simulink model "grav"  (R2017b)
settings: Solver=ode5  StartTime=0.0  StopTime=5*86400  FixedStep=60  RelTol=1e-3
undefined symbols (not defined in the file): Cube, G
settings Model: Creator=hazr_sh  LastModifiedBy=shriyahazra

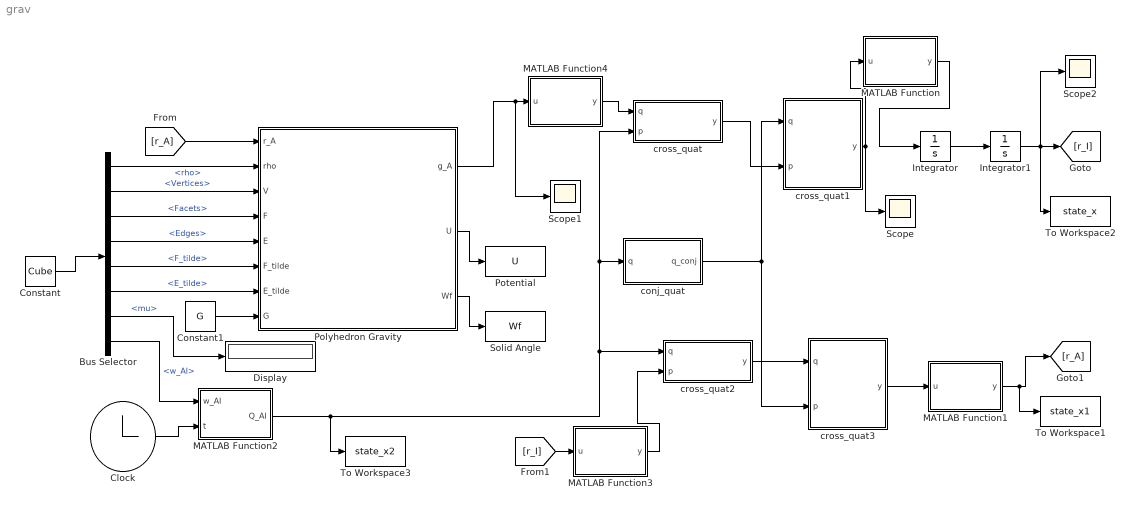
== system grav ==
  Bus Selector : BusSelector  OutputSignals=rho,Polyhedron.Vertices,Polyhedron.Facets,Polyhedron.Edges,Polyhedron.F_tilde,Polyhedron.E_tilde,mu,w_AI
  Clock : Clock
  Constant : Constant  Value=Cube  VectorParams1D=off  OutDataTypeStr=Bus: slBus1
  Constant1 : Constant  Value=G
  Display : Display
  Integrator : Integrator  InitialCondition=[100;100;0.1]
  Integrator1 : Integrator  InitialCondition=[80e3;60e3;50e3]
  MATLAB Function : MATLAB Function  TreatAsAtomicUnit=on
  MATLAB Function1 : MATLAB Function  TreatAsAtomicUnit=on
  MATLAB Function2 : MATLAB Function  TreatAsAtomicUnit=on
  MATLAB Function3 : MATLAB Function  TreatAsAtomicUnit=on
  MATLAB Function4 : MATLAB Function  TreatAsAtomicUnit=on
  Polyhedron Gravity : MATLAB Function  TreatAsAtomicUnit=on
  Potential : ToWorkspace  VariableName=U  SaveFormat=Timeseries  SampleTime=-1
  Scope : Scope
  Scope1 : Scope
  Scope2 : Scope
  Solid Angle : ToWorkspace  VariableName=Wf  SaveFormat=Timeseries  SampleTime=-1
  To Workspace1 : ToWorkspace  VariableName=state_x1  SampleTime=-1
  To Workspace2 : ToWorkspace  VariableName=state_x  SampleTime=-1
  To Workspace3 : ToWorkspace  VariableName=state_x2  SampleTime=-1
  conj_quat : MATLAB Function  TreatAsAtomicUnit=on
  cross_quat : MATLAB Function  TreatAsAtomicUnit=on
  cross_quat1 : MATLAB Function  TreatAsAtomicUnit=on
  cross_quat2 : MATLAB Function  TreatAsAtomicUnit=on
  cross_quat3 : MATLAB Function  TreatAsAtomicUnit=on
  wires:
  Bus Selector/3 -> Polyhedron Gravity/4(F)  "<Facets>"
  Bus Selector/7 -> Display/1  "<mu>"
  Constant1/1 -> Polyhedron Gravity/8(G)
  Constant/1 -> Bus Selector/1
  Polyhedron Gravity/3(Wf) -> Solid Angle/1
  Bus Selector/2 -> Polyhedron Gravity/3(V)  "<Vertices>"
  Bus Selector/5 -> Polyhedron Gravity/6(F_tilde)  "<F_tilde>"
  Bus Selector/4 -> Polyhedron Gravity/5(E)  "<Edges>"
  Bus Selector/6 -> Polyhedron Gravity/7(E_tilde)  "<E_tilde>"
  Polyhedron Gravity/2(U) -> Potential/1
  Bus Selector/1 -> Polyhedron Gravity/2(rho)  "<rho>"
  Integrator/1 -> Integrator1/1
  Polyhedron Gravity/1(g_A) -> Scope1/1, MATLAB Function4/1(u)
  cross_quat1/1(y) -> MATLAB Function/1(u), Scope/1
  Clock/1 -> MATLAB Function2/2(t)
  Integrator1/1 -> To Workspace2/1, Scope2/1, [r_I]
  [r_A] -> Polyhedron Gravity/1(r_A)
  [r_I] -> MATLAB Function3/1(u)
  cross_quat3/1(y) -> MATLAB Function1/1(u)
  Bus Selector/8 -> MATLAB Function2/1(w_AI)  "<w_AI>"
  MATLAB Function2/1(Q_AI) -> To Workspace3/1, cross_quat/2(p), conj_quat/1(q), cross_quat2/1(q)
  MATLAB Function4/1(y) -> cross_quat/1(q)
  conj_quat/1(q_conj) -> cross_quat3/2(p), cross_quat1/1(q)
  cross_quat/1(y) -> cross_quat1/2(p)
  cross_quat2/1(y) -> cross_quat3/1(q)
  MATLAB Function/1(y) -> Integrator/1
  MATLAB Function3/1(y) -> cross_quat2/2(p)
  MATLAB Function1/1(y) -> To Workspace1/1, [r_A]

== matlab function grav/cross_quat2 ==
  data: q input; y output; p input
function y = cross_quat(q, p)
% Quaternion Cross Product

q4= q(4);
p4= p(4);

q_vect= q(1:3);
p_vect= p(1:3);

y = [q4.*p_vect + p4.*q_vect - cross(q_vect, p_vect); q4*p4 - dot(q_vect,p_vect)];
end

== matlab function grav/MATLAB Function2 ==
  data: w_AI input; Q_AI output; t input
function Q_AI = fcn(w_AI,t)

Q_AI = [0; 0; sin(w_AI(3)*t/2); cos(w_AI(3)*t/2)];

end

== matlab function grav/cross_quat1 ==
  data: q input; y output; p input
function y = cross_quat(q, p)
% Quaternion Cross Product

q4= q(4);
p4= p(4);

q_vect= q(1:3);
p_vect= p(1:3);

y = [q4.*p_vect + p4.*q_vect - cross(q_vect, p_vect); q4*p4 - dot(q_vect,p_vect)];
end

== matlab function grav/conj_quat ==
  data: q input; q_conj output
function q_conj = conj_quat(q)
%Unit quaternion conjugation

q0= q(4);
q_vect= q(1:3);

q_conj = [-q_vect; q0];
end

== matlab function grav/cross_quat3 ==
  data: q input; y output; p input
function y = cross_quat(q, p)
% Quaternion Cross Product

q4= q(4);
p4= p(4);

q_vect= q(1:3);
p_vect= p(1:3);

y = [q4.*p_vect + p4.*q_vect - cross(q_vect, p_vect); q4*p4 - dot(q_vect,p_vect)];
end

== matlab function grav/cross_quat ==
  data: q input; y output; p input
function y = cross_quat(q, p)
% Quaternion Cross Product

q4= q(4);
p4= p(4);

q_vect= q(1:3);
p_vect= p(1:3);

y = [q4.*p_vect + p4.*q_vect - cross(q_vect, p_vect); q4*p4 - dot(q_vect,p_vect)];
end

== matlab function grav/MATLAB Function ==
  data: u input; y output
function y = fcn(u)
    y = [u(1); u(2); u(3)];
end

== matlab function grav/MATLAB Function1 ==
  data: u input; y output
function y = fcn(u)
    y = [u(1); u(2); u(3)];
end

== matlab function grav/MATLAB Function3 ==
  data: u input; y output
function y = fcn(u)
y =[u(1);u(2);u(3);0 ];
end

== matlab function grav/MATLAB Function4 ==
  data: u input; y output
function y = fcn(u)
y =[u(1);u(2);u(3);0 ];
end

== matlab function grav/Polyhedron Gravity ==
  data: r_A input; rho input; V input; F input; E input; F_tilde input; E_tilde input; g_A output; G input; U output; Wf output
function [g_A, U, Wf] = Poly_gravity(r_A,rho,V,F,E,F_tilde,E_tilde,G)
%% Function to calculate Cube gravity from Asteroid structure (from Get_Asteroid function)
%
% Inputs: r_A - position of a field point in Asteroid frame
%         Asteroid - Asteroid structure
%
% Outputs: g_A - gravitational acceleration in Asteroid frame
%          U - gravitational potential in Asteroid frame
%          Wf - THE solid angle, which shows whether the point is in or out
%               It can be used for stopping simulation if SC crashes

%% Initialization

Wf = 0;

Facets = [0 0 0]';
Edges = [0 0 0]';

U_edg = 0;
U_fac = 0;

S = r_A;

for j=1:1:size(E,1)
    
    % Calculate gravity due to edge potential
    
    R1 = V(E(j,1),:);    
    R2 = V(E(j,2),:);    

    Ri = R1'-S;
    ri = norm(Ri);
    
    Rj = R2'-S;
    rj = norm(Rj);
        
    Rij = Rj-Ri;
    eij = norm(Rij);

    Re1 =(Ri+Rj)/2;
   
    Le = log((ri+rj+eij)/(ri+rj-eij));
    
    if Le == Inf
     
        Le = 0;
     
    end
    
    Edges = (Le*E_tilde(:,:,j)*Re1)+Edges;
    U_edg = (Le*Re1'*E_tilde(:,:,j)*Re1)+U_edg;
    
end

 for i=1:1:(size(F,1))
    
    % Calculate gravity due to face potential
    
    R1 = V(F(i,1),:);    
    R2 = V(F(i,2),:);    
    R3 = V(F(i,3),:);
    

    Ri = R1'-S;
    ri = norm(Ri);
    
    Rj = R2'-S;
    rj = norm(Rj);
    
    Rk = R3'-S;
    rk = norm(Rk);
    
    
    wf = 2*atan2(dot(Ri, cross(Rj,Rk)),(ri*rj*rk+ri*dot(Rj,Rk)+rj*dot(Rk,Ri)+rk*dot(Ri,Rj)));
    
    Rf =(Ri+Rj+Rk)/3;

    U_fac = wf*Rf'*F_tilde(:,:,i)*Rf+U_fac;
    Facets = wf*F_tilde(:,:,i)*Rf+Facets;
    
    Wf = wf+Wf;
  
 end

g_A = G*rho*(-Edges+Facets);

U = 0.5*G*rho*(U_edg-U_fac);

end
